simulink model "mag_field_approx"  (R2016b)
settings: Solver=VariableStepAuto  StartTime=0.0  StopTime=10800  RelTol=1e-3
values from neighbouring files (symbols this model uses):
  fsw_params = init_fsw_params()    [mag_vec_approx_test_init.m]
libraries: GPS_time_lib x1, mag_vec_lib x1, sgp4_lib_fsw x1, time_coord_rotation_lib x1
settings Model: Creator=taylorreynolds  LastModifiedBy=taylorreynolds

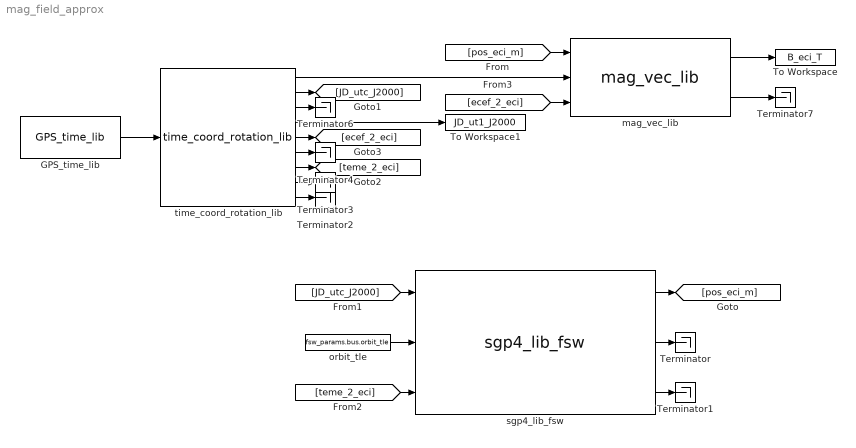
== system mag_field_approx ==
  GPS_time_lib : GPS_time_lib/GPS_time_lib
  Terminator{,1..4,6..7} (7 alike) : Terminator
  To Workspace : ToWorkspace  VariableName=B_eci_T  SaveFormat=Timeseries  SampleTime=-1
  To Workspace1 : ToWorkspace  VariableName=JD_ut1_J2000  SaveFormat=Timeseries  SampleTime=-1
  mag_vec_lib : mag_vec_lib/mag_vec_lib
  orbit_tle : Constant  Value=fsw_params.bus.orbit_tle
  sgp4_lib_fsw : sgp4_lib_fsw/sgp4_lib_fsw
  time_coord_rotation_lib : time_coord_rotation_lib/time_coord_rotation_lib
  wires:
  GPS_time_lib/1 -> time_coord_rotation_lib/1
  sgp4_lib_fsw/1 -> [pos_eci_m]
  [pos_eci_m] -> mag_vec_lib/1
  time_coord_rotation_lib/2 -> [JD_utc_J2000]
  [JD_utc_J2000] -> sgp4_lib_fsw/1
  time_coord_rotation_lib/7 -> [teme_2_eci]
  [teme_2_eci] -> sgp4_lib_fsw/3
  time_coord_rotation_lib/5 -> [ecef_2_eci]
  time_coord_rotation_lib/1 -> mag_vec_lib/2
  [ecef_2_eci] -> mag_vec_lib/3
  orbit_tle/1 -> sgp4_lib_fsw/2
  sgp4_lib_fsw/2 -> Terminator/1
  sgp4_lib_fsw/3 -> Terminator1/1
  time_coord_rotation_lib/9 -> Terminator2/1
  time_coord_rotation_lib/8 -> Terminator3/1
  time_coord_rotation_lib/6 -> Terminator4/1
  time_coord_rotation_lib/4 -> To Workspace1/1
  time_coord_rotation_lib/3 -> Terminator6/1
  mag_vec_lib/2 -> Terminator7/1
  mag_vec_lib/1 -> To Workspace/1
